simulink model "finetuning"  (R2020b)
settings: Solver=ode45  StartTime=0.0  StopTime=8  MaxStep=0.000002  RelTol=1e-3
libraries: simulink x4, simulink_extras x4
settings Model: Creator=Ocean  LastModifiedBy=Somith Das

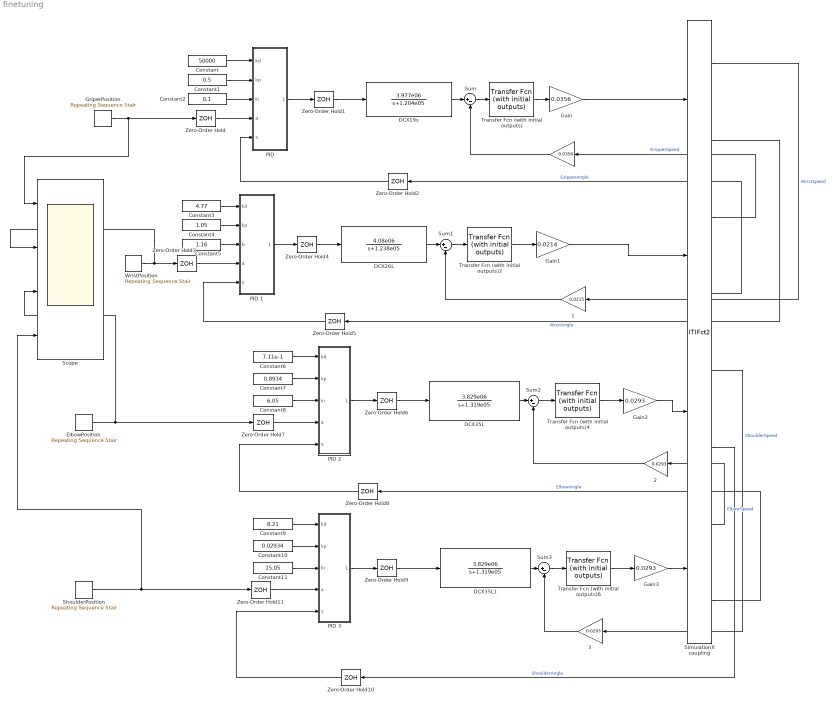
== system finetuning ==
  " " : Gain  Gain=0.0356
  " 1" : Gain  Gain=0.0215
  " 2" : Gain  Gain=0.0293
  " 3" : Gain  Gain=0.0293
  Constant : Constant  Value=50000
  Constant1 : Constant  Value=0.5
  Constant10 : Constant  Value=0.02934
  Constant11 : Constant  Value=15.05
  Constant2 : Constant  Value=0.1
  Constant3 : Constant  Value=4.77
  Constant4 : Constant  Value=1.05
  Constant5 : Constant  Value=1.16
  Constant6 : Constant  Value=7.11e-1
  Constant7 : Constant  Value=0.8934
  Constant8 : Constant  Value=6.05
  Constant9 : Constant  Value=8.21
  DCX19s : TransferFcn  Numerator=[3.977e06]  Denominator=[1 1.204e05]
  DCX26L : TransferFcn  Numerator=[4.08e06]  Denominator=[1 1.238e05]
  DCX35L : TransferFcn  Numerator=[3.829e06]  Denominator=[1 1.319e05]
  DCX35L1 : TransferFcn  Numerator=[3.829e06]  Denominator=[1 1.319e05]
  ElbowPosition : simulink/Sources/Repeating Sequence Stair  OutValues="[0 0/180*pi 0/180*pi      10/180*pi 20/180*pi 30/180*pi 40/180*pi 50/180*pi 50/180*pi 50/180*pi 50/180*pi 50/180*pi 50/180*pi 40/180*pi 30/180*pi 20/180*pi 10/180*pi 0 0/180*pi 0/180*pi 0 0/180*pi 0/180*pi   10/180*pi  15/180*pi  20/180*pi 25/180*pi 30/180*pi 30/180*pi  30/180*pi 30/180*pi 30/180*pi 30/180*pi 25/180*pi 20/180*pi 15/180*pi 10/180*pi 0/180*pi 0/180*pi 0/180*pi].'"  tsamp=0.2  OutMin=[]  OutMax=[]  OutDataTypeStr=double  OutputDataTypeScalingMode=double  OutDataType=fixdt(0,8)  ConRadixGroup=Best Precision: Vector-wise  OutScaling=2^-12
  Gain : Gain  Gain=0.0356
  Gain1 : Gain  Gain=0.0214
  Gain2 : Gain  Gain=0.0293
  Gain3 : Gain  Gain=0.0293
  GriperPosition : simulink/Sources/Repeating Sequence Stair  OutValues="[0 -20/180*pi -20/180*pi -20/180*pi 0/180*pi   0/180*pi   0/180*pi  0/180*pi 0/180*pi -33/180*pi -33/180*pi -33/180*pi  -33/180*pi  -33/180*pi -33/180*pi -33/180*pi -33/180*pi -33/180*pi -33/180*pi -33/180*pi -33/180*pi -33/180*pi -33/180*pi -33/180*pi -33/180*pi   -33/180*pi   -33/180*pi  0/180*pi 0/180*pi 0/180*pi 0/180*pi 0/180*pi 0/180*pi 0/180*pi 0/180*pi 0/180*pi 0/180*pi 0/180*pi   0/180*pi  0/180*pi].'"  tsamp=0.2  OutMin=[]  OutMax=[]  OutDataTypeStr=double  OutputDataTypeScalingMode=double  OutDataType=fixdt(0,8)  ConRadixGroup=Best Precision: Vector-wise  OutScaling=2^-12
  "PID " : MATLAB Function  TreatAsAtomicUnit=on
  PID 1 : MATLAB Function  TreatAsAtomicUnit=on
  PID 2 : MATLAB Function  TreatAsAtomicUnit=on
  PID 3 : MATLAB Function  TreatAsAtomicUnit=on
  Scope : Scope  NumInputPorts=4
  ShoulderPosition : simulink/Sources/Repeating Sequence Stair  OutValues=[0 10/180*pi 20/180*pi 30/180*pi 35/180*pi 35/180*pi 35/180*pi 35/180*pi 35/180*pi 35/180*pi 35/180*pi 35/180*pi 35/180*pi 35/180*pi 35/180*pi 35/180*pi 30/180*pi 20/180*pi 10/180*pi 0 0 -10/180*pi -20/180*pi -30/180*pi -40/180*pi -50/180*pi -60/180*pi -60/180*pi -60/180*pi -60/180*pi -60/180*pi -60/180*pi -60/180*pi -60/180*pi -50/180*pi -40/180*pi -30/180*pi -20/180*pi -10/180*pi 0].'  tsamp=0.2  OutMin=[]  OutMax=[]  OutDataTypeStr=double  OutputDataTypeScalingMode=double  OutDataType=fixdt(0,8)  ConRadixGroup=Best Precision: Vector-wise  OutScaling=2^-12
  SimulationX coupling : S-Function  FunctionName=ITIFct2  Parameters=ip, port, ts, nIn, nOut  SFunctionDeploymentMode=off  EnableBusSupport=off  mask{ip='localhost', port=2048, ts=0.001, nIn=4, nOut=8}
      mask prompts: ip "Address: ip"; port "Port Number: port [-]"; ts "Communication Step Size: ts [s]"; nIn "Input Vector Dimension (to SimulationX): nIn [-]"; nOut "Output Vector Dimension (from SimulationX): nOut [-]"
      mask help: Coupling Element
  Sum{,1..3} (4 alike) : Sum  Inputs=|+-
  Transfer Fcn (with initial outputs) : simulink_extras/Additional Linear/Transfer Fcn (with initial outputs)  N=[1]  D="[0.0013  22.8]"  Y0=0  U0=0
  Transfer Fcn (with initial outputs)2 : simulink_extras/Additional Linear/Transfer Fcn (with initial outputs)  N=[1]  D="[1.2900e-04  0.74]"  Y0=0  U0=0
  Transfer Fcn (with initial outputs)4 : simulink_extras/Additional Linear/Transfer Fcn (with initial outputs)  N=[1]  D="[1.2100e-04  0.346]"  Y0=0  U0=0
  Transfer Fcn (with initial outputs)6 : simulink_extras/Additional Linear/Transfer Fcn (with initial outputs)  N=[1]  D="[1.2100e-04  0.346]"  Y0=0  U0=0
  WristPosition : simulink/Sources/Repeating Sequence Stair  OutValues="[0 0/180*pi 0/180*pi   -10/180*pi -20/180*pi -30/180*pi -40/180*pi -50/180*pi -50/180*pi -50/180*pi -50/180*pi -50/180*pi -50/180*pi -40/180*pi -30/180*pi -20/180*pi -10/180*pi 0 0/180*pi -10/180*pi   -20/180*pi -30/180*pi  -40/180*pi   -50/180*pi   -50/180*pi  -50/180*pi  -50/180*pi -50/180*pi   -50/180*pi  -50/180*pi  -50/180*pi -40/180*pi -30/180*pi -20/180*pi -10/180*pi 0 0].'"  tsamp=0.2  OutMin=[]  OutMax=[]  OutDataTypeStr=double  OutputDataTypeScalingMode=double  OutDataType=fixdt(0,8)  ConRadixGroup=Best Precision: Vector-wise  OutScaling=2^-12
  Zero-Order Hold{,1..11} (12 alike) : ZeroOrderHold  SampleTime=0.00002
  wires:
  Constant/1 -> "PID "/1(kd)
  Constant1/1 -> "PID "/2(kp)
  Constant2/1 -> "PID "/3(ki)
  Transfer Fcn (with initial outputs)/1 -> Gain/1
  Sum/1 -> Transfer Fcn (with initial outputs)/1
  DCX19s/1 -> Sum/1
  " "/1 -> Sum/2
  Constant3/1 -> PID 1/1(kd)
  Constant4/1 -> PID 1/2(kp)
  Constant5/1 -> PID 1/3(ki)
  Transfer Fcn (with initial outputs)2/1 -> Gain1/1
  Sum1/1 -> Transfer Fcn (with initial outputs)2/1
  DCX26L/1 -> Sum1/1
  " 1"/1 -> Sum1/2
  Constant6/1 -> PID 2/1(kd)
  Constant7/1 -> PID 2/2(kp)
  Constant8/1 -> PID 2/3(ki)
  Transfer Fcn (with initial outputs)4/1 -> Gain2/1
  PID 2/1(output) -> Zero-Order Hold6/1
  Sum2/1 -> Transfer Fcn (with initial outputs)4/1
  DCX35L/1 -> Sum2/1
  " 2"/1 -> Sum2/2
  Constant11/1 -> PID 3/3(ki)
  Transfer Fcn (with initial outputs)6/1 -> Gain3/1
  Sum3/1 -> Transfer Fcn (with initial outputs)6/1
  DCX35L1/1 -> Sum3/1
  Constant9/1 -> PID 3/1(kd)
  Constant10/1 -> PID 3/2(kp)
  Gain/1 -> SimulationX coupling/1
  Gain1/1 -> SimulationX coupling/2
  Gain2/1 -> SimulationX coupling/3
  Gain3/1 -> SimulationX coupling/4
  SimulationX coupling/6 -> Zero-Order Hold10/1  "ShoulderAngle"
  SimulationX coupling/7 -> " 2"/1  "ElbowSpeed"
  SimulationX coupling/8 -> Zero-Order Hold8/1  "ElbowAngle"
  SimulationX coupling/2 -> Zero-Order Hold5/1  "WristAngle"
  SimulationX coupling/1 -> " 1"/1  "WristSpeed"
  SimulationX coupling/3 -> " "/1  "GripperSpeed"
  SimulationX coupling/4 -> Zero-Order Hold2/1  "GripperAngle"
  SimulationX coupling/5 -> " 3"/1  "ShoulderSpeed"
  " 3"/1 -> Sum3/2
  Zero-Order Hold/1 -> "PID "/4(desiredPos)
  Zero-Order Hold1/1 -> DCX19s/1
  "PID "/1(output) -> Zero-Order Hold1/1
  Zero-Order Hold2/1 -> "PID "/5(actualPos)
  Zero-Order Hold3/1 -> PID 1/4(desiredPos)
  PID 1/1(output) -> Zero-Order Hold4/1
  Zero-Order Hold4/1 -> DCX26L/1
  Zero-Order Hold5/1 -> PID 1/5(actualPos)
  Zero-Order Hold6/1 -> DCX35L/1
  Zero-Order Hold7/1 -> PID 2/4(desiredPos)
  Zero-Order Hold8/1 -> PID 2/5(actualPos)
  PID 3/1(output) -> Zero-Order Hold9/1
  Zero-Order Hold9/1 -> DCX35L1/1
  Zero-Order Hold10/1 -> PID 3/5(actualPos)
  Zero-Order Hold11/1 -> PID 3/4(desiredPos)
  GriperPosition/1 -> Scope/1, Zero-Order Hold/1
  ShoulderPosition/1 -> Scope/4, Zero-Order Hold11/1
  ElbowPosition/1 -> Scope/3, Zero-Order Hold7/1
  WristPosition/1 -> Scope/2, Zero-Order Hold3/1

== matlab function finetuning/PID 1 ==
  settings: updateMethod=DISCRETE  sampleTime=0.00002
  data: kd input; kp input; output output; ki input; desiredPos input; actualPos input
function output = fcn(kd,kp,ki,desiredPos,actualPos)
n = 6;
cf = 50000;
period = 1/cf;
p = 4*cf/n;


persistent prevError
if isempty(prevError)
    prevError = 0;
end

%prop calc
error = desiredPos - actualPos;

%integral calc
integral = period*(error+prevError)/2;

%derivative calc

ept = zeros(1,n);
for i = 1:n
    ept(i) = exp(-p*i*period); 
end

persistent signal
if isempty(signal)
    signal = zeros(1,n);
end

signal(1) = (error-prevError)/period;
derivative = dot(signal,ept);

for i = 1:n-1
    signal(n+1-i) = signal(n-i);
end

output = kp*error + ki*integral + kd*derivative;
prevError = error;
end


%typical values in kHz range for delta t

== matlab function finetuning/PID  ==
  settings: updateMethod=DISCRETE  sampleTime=0.00002
  data: kd input; kp input; output output; ki input; desiredPos input; actualPos input
function output = fcn(kd,kp,ki,desiredPos,actualPos)
n = 6;
cf = 50000;
period = 1/cf;
p = 4*cf/n;


persistent prevError
if isempty(prevError)
    prevError = 0;
end

%prop calc
error = desiredPos - actualPos;

%integral calc
integral = period*(error+prevError)/2;

%derivative calc

ept = zeros(1,n);
for i = 1:n
    ept(i) = exp(-p*i*period); 
end

persistent signal
if isempty(signal)
    signal = zeros(1,n);
end

signal(1) = (error-prevError)/period;
derivative = dot(signal,ept);

for i = 1:n-1
    signal(n+1-i) = signal(n-i);
end

output = kp*error + ki*integral + kd*derivative;
prevError = error;
end


%typical values in kHz range for delta t

== matlab function finetuning/PID 2 ==
  settings: updateMethod=DISCRETE  sampleTime=0.00002
  data: kd input; kp input; output output; ki input; desiredPos input; actualPos input
function output = fcn(kd,kp,ki,desiredPos,actualPos)
n = 6;
cf = 50000;
period = 1/cf;
p = 4*cf/n;


persistent prevError
if isempty(prevError)
    prevError = 0;
end

%prop calc
error = desiredPos - actualPos;

%integral calc
integral = period*(error+prevError)/2;

%derivative calc

ept = zeros(1,n);
for i = 1:n
    ept(i) = exp(-p*i*period); 
end

persistent signal
if isempty(signal)
    signal = zeros(1,n);
end

signal(1) = (error-prevError)/period;
derivative = dot(signal,ept);

for i = 1:n-1
    signal(n+1-i) = signal(n-i);
end

output = kp*error + ki*integral + kd*derivative;
prevError = error;
end


%typical values in kHz range for delta t

== matlab function finetuning/PID 3 ==
  settings: updateMethod=DISCRETE  sampleTime=0.00002
  data: kd input; kp input; output output; ki input; desiredPos input; actualPos input
function output = fcn(kd,kp,ki,desiredPos,actualPos)
n = 6;
cf = 50000;
period = 1/cf;
p = 4*cf/n;


persistent prevError
if isempty(prevError)
    prevError = 0;
end

%prop calc
error = desiredPos - actualPos;

%integral calc
integral = period*(error+prevError)/2;

%derivative calc

ept = zeros(1,n);
for i = 1:n
    ept(i) = exp(-p*i*period); 
end

persistent signal
if isempty(signal)
    signal = zeros(1,n);
end

signal(1) = (error-prevError)/period;
derivative = dot(signal,ept);

for i = 1:n-1
    signal(n+1-i) = signal(n-i);
end

output = kp*error + ki*integral + kd*derivative;
prevError = error;
end


%typical values in kHz range for delta t
